simulink model "Model"  (R2020b)
settings: Solver=FixedStepDiscrete  StartTime=0.0  StopTime=inf  RelTol=1e-3
undefined symbols (not defined in the file): C12, designMultirateFIR, dt0
libraries: dspmlti4 x96, dspsrcs4 x89
(part 1 of 6)
settings Model: Creator=User  LastModifiedBy=User

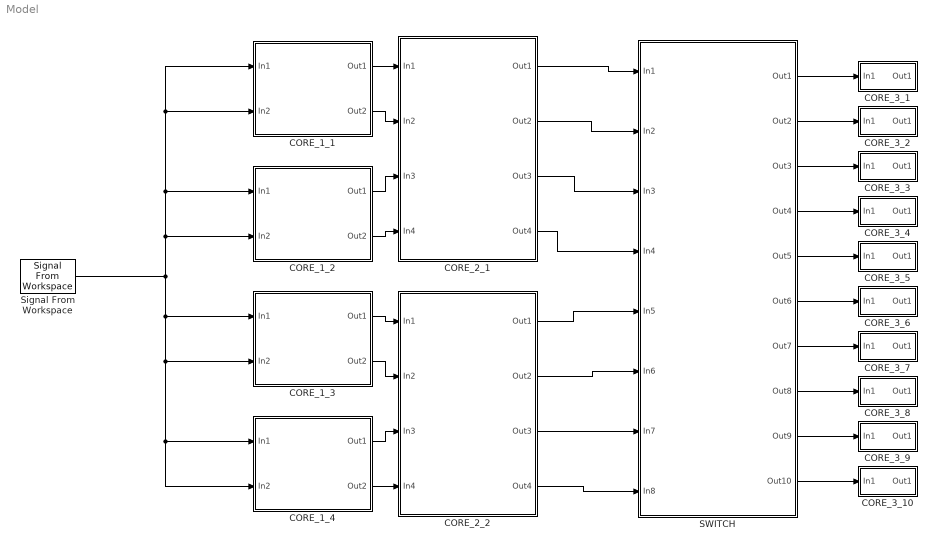
== system Model ==
  CORE_1_1 : Subsystem
  CORE_1_2 : Subsystem
  CORE_1_3 : Subsystem
  CORE_1_4 : Subsystem
  CORE_2_1 : Subsystem
  CORE_2_2 : Subsystem
  CORE_3_1 : Subsystem
  CORE_3_10 : Subsystem
  CORE_3_2 : Subsystem
  CORE_3_3 : Subsystem
  CORE_3_4 : Subsystem
  CORE_3_5 : Subsystem
  CORE_3_6 : Subsystem
  CORE_3_7 : Subsystem
  CORE_3_8 : Subsystem
  CORE_3_9 : Subsystem
  SWITCH : Subsystem
  Signal From Workspace : dspsrcs4/Signal From Workspace  X=x  Ts=dt0  nsamps=1  OutputAfterFinalValue=Cyclic repetition  ignoreOrWarnInputAndFrameLengths=off  OutputFrames=off
  wires:
  CORE_1_4/1(Out1) -> CORE_2_2/3(In3)
  CORE_1_4/2(Out2) -> CORE_2_2/4(In4)
  Signal From Workspace/1 -> CORE_1_2/2(In2), CORE_1_2/1(In1), CORE_1_1/2(In2), CORE_1_1/1(In1), CORE_1_3/1(In1), CORE_1_3/2(In2), CORE_1_4/1(In1), CORE_1_4/2(In2)
  CORE_1_3/2(Out2) -> CORE_2_2/2(In2)
  CORE_1_3/1(Out1) -> CORE_2_2/1(In1)
  CORE_1_1/1(Out1) -> CORE_2_1/1(In1)
  CORE_1_1/2(Out2) -> CORE_2_1/2(In2)
  CORE_1_2/1(Out1) -> CORE_2_1/3(In3)
  CORE_1_2/2(Out2) -> CORE_2_1/4(In4)
  CORE_2_1/1(Out1) -> SWITCH/1(In1)
  CORE_2_1/2(Out2) -> SWITCH/2(In2)
  CORE_2_1/3(Out3) -> SWITCH/3(In3)
  CORE_2_1/4(Out4) -> SWITCH/4(In4)
  CORE_2_2/1(Out1) -> SWITCH/5(In5)
  CORE_2_2/2(Out2) -> SWITCH/6(In6)
  CORE_2_2/3(Out3) -> SWITCH/7(In7)
  CORE_2_2/4(Out4) -> SWITCH/8(In8)
  SWITCH/1(Out1) -> CORE_3_1/1(In1)
  SWITCH/2(Out2) -> CORE_3_2/1(In1)
  SWITCH/3(Out3) -> CORE_3_3/1(In1)
  SWITCH/6(Out6) -> CORE_3_6/1(In1)
  SWITCH/5(Out5) -> CORE_3_5/1(In1)
  SWITCH/4(Out4) -> CORE_3_4/1(In1)
  SWITCH/9(Out9) -> CORE_3_9/1(In1)
  SWITCH/8(Out8) -> CORE_3_8/1(In1)
  SWITCH/7(Out7) -> CORE_3_7/1(In1)
  SWITCH/10(Out10) -> CORE_3_10/1(In1)

== system Model/CORE_1_1 ==
  In1 : Inport
  In2 : Inport  Port=2
  Complex to Real-Imag{,1..3} (4 alike) : ComplexToRealImag
  Constant : Constant  Value=C12  SampleTime=dt0
  Constant1 : Constant  Value=C12  SampleTime=dt0
  DDS_Gen1 : Subsystem
  DDS_Gen2 : Subsystem
  FIR Dec1 : dspmlti4/FIR Decimation  FilterSource=Input port  h=designMultirateFIR(1,2)  D=2  filtStruct=Direct form  FilterObject=FDECIM  framing=Allow multirate processing  inputOffset=0  outputBufInitCond=0  roundingMode=Floor  overflowMode=off  firstCoeffDataTypeStr=Inherit: Same word length as input  firstCoeffMin=[]  firstCoeffMax=[]  firstCoeffLastDataTypeStr=Inherit: Same word length as input  outputDataTypeStr=Inherit: Same as accumulator  outputMin=[]  outputMax=[]  outputLastDataTypeStr=Inherit: Same as accumulator
  FIR Dec2 : dspmlti4/FIR Decimation  FilterSource=Input port  h=designMultirateFIR(1,2)  D=2  filtStruct=Direct form  FilterObject=FDECIM  framing=Allow multirate processing  inputOffset=0  outputBufInitCond=0  roundingMode=Floor  overflowMode=off  firstCoeffDataTypeStr=Inherit: Same word length as input  firstCoeffMin=[]  firstCoeffMax=[]  firstCoeffLastDataTypeStr=Inherit: Same word length as input  outputDataTypeStr=Inherit: Same as accumulator  outputMin=[]  outputMax=[]  outputLastDataTypeStr=Inherit: Same as accumulator
  Freq1 : Constant  Value=-17.5e6
  Freq2 : Constant  Value=-12.5e6
  Mixer1 : Subsystem
  Mixer2 : Subsystem
  Real-Imag to Complex : RealImagToComplex
  Real-Imag to Complex1 : RealImagToComplex
  Out1 : Outport
  Out2 : Outport  Port=2
  wires:
  Complex to Real-Imag/1 -> Mixer1/1(Input_I)
  Complex to Real-Imag/2 -> Mixer1/2(Input_Q)
  Constant1/1 -> FIR Dec2/2
  Mixer2/2(Output_Q) -> Real-Imag to Complex1/2
  Mixer2/1(Output_I) -> Real-Imag to Complex1/1
  Complex to Real-Imag2/1 -> Mixer2/1(Input_I)
  Mixer1/2(Output_Q) -> Real-Imag to Complex/2
  Complex to Real-Imag2/2 -> Mixer2/2(Input_Q)
  Complex to Real-Imag3/1 -> Mixer2/3(DDS_I)
  FIR Dec2/1 -> Out2/1
  Complex to Real-Imag1/1 -> Mixer1/3(DDS_I)
  DDS_Gen1/1(Out1) -> Complex to Real-Imag1/1
  Freq1/1 -> DDS_Gen1/1(In1)
  Complex to Real-Imag1/2 -> Mixer1/4(DDS_Q)
  Real-Imag to Complex1/1 -> FIR Dec2/1
  Complex to Real-Imag3/2 -> Mixer2/4(DDS_Q)
  Freq2/1 -> DDS_Gen2/1(In1)
  DDS_Gen2/1(Out1) -> Complex to Real-Imag3/1
  Real-Imag to Complex/1 -> FIR Dec1/1
  Mixer1/1(Output_I) -> Real-Imag to Complex/1
  Constant/1 -> FIR Dec1/2
  In2/1 -> Complex to Real-Imag2/1
  FIR Dec1/1 -> Out1/1
  In1/1 -> Complex to Real-Imag/1

== system Model/CORE_1_2 ==
  In1 : Inport
  In2 : Inport  Port=2
  Complex to Real-Imag{,1..3} (4 alike) : ComplexToRealImag
  Constant : Constant  Value=C12  SampleTime=dt0
  Constant1 : Constant  Value=C12  SampleTime=dt0
  DDS_Gen1 : Subsystem
  DDS_Gen2 : Subsystem
  FIR Dec1 : dspmlti4/FIR Decimation  FilterSource=Input port  h=designMultirateFIR(1,2)  D=2  filtStruct=Direct form  FilterObject=FDECIM  framing=Allow multirate processing  inputOffset=0  outputBufInitCond=0  roundingMode=Floor  overflowMode=off  firstCoeffDataTypeStr=Inherit: Same word length as input  firstCoeffMin=[]  firstCoeffMax=[]  firstCoeffLastDataTypeStr=Inherit: Same word length as input  outputDataTypeStr=Inherit: Same as accumulator  outputMin=[]  outputMax=[]  outputLastDataTypeStr=Inherit: Same as accumulator
  FIR Dec2 : dspmlti4/FIR Decimation  FilterSource=Input port  h=designMultirateFIR(1,2)  D=2  filtStruct=Direct form  FilterObject=FDECIM  framing=Allow multirate processing  inputOffset=0  outputBufInitCond=0  roundingMode=Floor  overflowMode=off  firstCoeffDataTypeStr=Inherit: Same word length as input  firstCoeffMin=[]  firstCoeffMax=[]  firstCoeffLastDataTypeStr=Inherit: Same word length as input  outputDataTypeStr=Inherit: Same as accumulator  outputMin=[]  outputMax=[]  outputLastDataTypeStr=Inherit: Same as accumulator
  Freq1 : Constant  Value=-7.5e6
  Freq2 : Constant  Value=-2.5e6
  Mixer1 : Subsystem
  Mixer2 : Subsystem
  Real-Imag to Complex : RealImagToComplex
  Real-Imag to Complex1 : RealImagToComplex
  Out1 : Outport
  Out2 : Outport  Port=2
  wires:
  Complex to Real-Imag/1 -> Mixer1/1(Input_I)
  Complex to Real-Imag/2 -> Mixer1/2(Input_Q)
  Constant1/1 -> FIR Dec2/2
  Mixer2/2(Output_Q) -> Real-Imag to Complex1/2
  Mixer2/1(Output_I) -> Real-Imag to Complex1/1
  Complex to Real-Imag2/1 -> Mixer2/1(Input_I)
  Mixer1/2(Output_Q) -> Real-Imag to Complex/2
  Complex to Real-Imag2/2 -> Mixer2/2(Input_Q)
  Complex to Real-Imag3/1 -> Mixer2/3(DDS_I)
  FIR Dec2/1 -> Out2/1
  Complex to Real-Imag1/1 -> Mixer1/3(DDS_I)
  DDS_Gen1/1(Out1) -> Complex to Real-Imag1/1
  Freq1/1 -> DDS_Gen1/1(In1)
  Complex to Real-Imag1/2 -> Mixer1/4(DDS_Q)
  Real-Imag to Complex1/1 -> FIR Dec2/1
  Complex to Real-Imag3/2 -> Mixer2/4(DDS_Q)
  Freq2/1 -> DDS_Gen2/1(In1)
  DDS_Gen2/1(Out1) -> Complex to Real-Imag3/1
  Real-Imag to Complex/1 -> FIR Dec1/1
  Mixer1/1(Output_I) -> Real-Imag to Complex/1
  Constant/1 -> FIR Dec1/2
  In2/1 -> Complex to Real-Imag2/1
  FIR Dec1/1 -> Out1/1
  In1/1 -> Complex to Real-Imag/1

== system Model/CORE_1_3 ==
  In1 : Inport
  In2 : Inport  Port=2
  Complex to Real-Imag{,1..3} (4 alike) : ComplexToRealImag
  Constant : Constant  Value=C12  SampleTime=dt0
  Constant1 : Constant  Value=C12  SampleTime=dt0
  DDS_Gen1 : Subsystem
  DDS_Gen2 : Subsystem
  FIR Dec1 : dspmlti4/FIR Decimation  FilterSource=Input port  h=designMultirateFIR(1,2)  D=2  filtStruct=Direct form  FilterObject=FDECIM  framing=Allow multirate processing  inputOffset=0  outputBufInitCond=0  roundingMode=Floor  overflowMode=off  firstCoeffDataTypeStr=Inherit: Same word length as input  firstCoeffMin=[]  firstCoeffMax=[]  firstCoeffLastDataTypeStr=Inherit: Same word length as input  outputDataTypeStr=Inherit: Same as accumulator  outputMin=[]  outputMax=[]  outputLastDataTypeStr=Inherit: Same as accumulator
  FIR Dec2 : dspmlti4/FIR Decimation  FilterSource=Input port  h=designMultirateFIR(1,2)  D=2  filtStruct=Direct form  FilterObject=FDECIM  framing=Allow multirate processing  inputOffset=0  outputBufInitCond=0  roundingMode=Floor  overflowMode=off  firstCoeffDataTypeStr=Inherit: Same word length as input  firstCoeffMin=[]  firstCoeffMax=[]  firstCoeffLastDataTypeStr=Inherit: Same word length as input  outputDataTypeStr=Inherit: Same as accumulator  outputMin=[]  outputMax=[]  outputLastDataTypeStr=Inherit: Same as accumulator
  Freq1 : Constant  Value=2.5e6
  Freq2 : Constant  Value=7.5e6
  Mixer1 : Subsystem
  Mixer2 : Subsystem
  Real-Imag to Complex : RealImagToComplex
  Real-Imag to Complex1 : RealImagToComplex
  Out1 : Outport
  Out2 : Outport  Port=2
  wires:
  Complex to Real-Imag/1 -> Mixer1/1(Input_I)
  Complex to Real-Imag/2 -> Mixer1/2(Input_Q)
  Constant1/1 -> FIR Dec2/2
  Mixer2/2(Output_Q) -> Real-Imag to Complex1/2
  Mixer2/1(Output_I) -> Real-Imag to Complex1/1
  Complex to Real-Imag2/1 -> Mixer2/1(Input_I)
  Mixer1/2(Output_Q) -> Real-Imag to Complex/2
  Complex to Real-Imag2/2 -> Mixer2/2(Input_Q)
  Complex to Real-Imag3/1 -> Mixer2/3(DDS_I)
  FIR Dec2/1 -> Out2/1
  Complex to Real-Imag1/1 -> Mixer1/3(DDS_I)
  DDS_Gen1/1(Out1) -> Complex to Real-Imag1/1
  Freq1/1 -> DDS_Gen1/1(In1)
  Complex to Real-Imag1/2 -> Mixer1/4(DDS_Q)
  Real-Imag to Complex1/1 -> FIR Dec2/1
  Complex to Real-Imag3/2 -> Mixer2/4(DDS_Q)
  Freq2/1 -> DDS_Gen2/1(In1)
  DDS_Gen2/1(Out1) -> Complex to Real-Imag3/1
  Real-Imag to Complex/1 -> FIR Dec1/1
  Mixer1/1(Output_I) -> Real-Imag to Complex/1
  Constant/1 -> FIR Dec1/2
  In2/1 -> Complex to Real-Imag2/1
  FIR Dec1/1 -> Out1/1
  In1/1 -> Complex to Real-Imag/1

== system Model/CORE_1_4 ==
  In1 : Inport
  In2 : Inport  Port=2
  Complex to Real-Imag{,1..3} (4 alike) : ComplexToRealImag
  Constant : Constant  Value=C12  SampleTime=dt0
  Constant1 : Constant  Value=C12  SampleTime=dt0
  DDS_Gen1 : Subsystem
  DDS_Gen2 : Subsystem
  FIR Dec1 : dspmlti4/FIR Decimation  FilterSource=Input port  h=designMultirateFIR(1,2)  D=2  filtStruct=Direct form  FilterObject=FDECIM  framing=Allow multirate processing  inputOffset=0  outputBufInitCond=0  roundingMode=Floor  overflowMode=off  firstCoeffDataTypeStr=Inherit: Same word length as input  firstCoeffMin=[]  firstCoeffMax=[]  firstCoeffLastDataTypeStr=Inherit: Same word length as input  outputDataTypeStr=Inherit: Same as accumulator  outputMin=[]  outputMax=[]  outputLastDataTypeStr=Inherit: Same as accumulator
  FIR Dec2 : dspmlti4/FIR Decimation  FilterSource=Input port  h=designMultirateFIR(1,2)  D=2  filtStruct=Direct form  FilterObject=FDECIM  framing=Allow multirate processing  inputOffset=0  outputBufInitCond=0  roundingMode=Floor  overflowMode=off  firstCoeffDataTypeStr=Inherit: Same word length as input  firstCoeffMin=[]  firstCoeffMax=[]  firstCoeffLastDataTypeStr=Inherit: Same word length as input  outputDataTypeStr=Inherit: Same as accumulator  outputMin=[]  outputMax=[]  outputLastDataTypeStr=Inherit: Same as accumulator
  Freq1 : Constant  Value=12.5e6
  Freq2 : Constant  Value=17.5e6
  Mixer1 : Subsystem
  Mixer2 : Subsystem
  Real-Imag to Complex : RealImagToComplex
  Real-Imag to Complex1 : RealImagToComplex
  Out1 : Outport
  Out2 : Outport  Port=2
  wires:
  Complex to Real-Imag/1 -> Mixer1/1(Input_I)
  Complex to Real-Imag/2 -> Mixer1/2(Input_Q)
  Constant1/1 -> FIR Dec2/2
  Mixer2/2(Output_Q) -> Real-Imag to Complex1/2
  Mixer2/1(Output_I) -> Real-Imag to Complex1/1
  Complex to Real-Imag2/1 -> Mixer2/1(Input_I)
  Mixer1/2(Output_Q) -> Real-Imag to Complex/2
  Complex to Real-Imag2/2 -> Mixer2/2(Input_Q)
  Complex to Real-Imag3/1 -> Mixer2/3(DDS_I)
  FIR Dec2/1 -> Out2/1
  Complex to Real-Imag1/1 -> Mixer1/3(DDS_I)
  DDS_Gen1/1(Out1) -> Complex to Real-Imag1/1
  Freq1/1 -> DDS_Gen1/1(In1)
  Complex to Real-Imag1/2 -> Mixer1/4(DDS_Q)
  Real-Imag to Complex1/1 -> FIR Dec2/1
  Complex to Real-Imag3/2 -> Mixer2/4(DDS_Q)
  Freq2/1 -> DDS_Gen2/1(In1)
  DDS_Gen2/1(Out1) -> Complex to Real-Imag3/1
  Real-Imag to Complex/1 -> FIR Dec1/1
  Mixer1/1(Output_I) -> Real-Imag to Complex/1
  Constant/1 -> FIR Dec1/2
  In2/1 -> Complex to Real-Imag2/1
  FIR Dec1/1 -> Out1/1
  In1/1 -> Complex to Real-Imag/1

== system Model/CORE_2_1 ==
  In1 : Inport
  In2 : Inport  Port=2
  In3 : Inport  Port=3
  In4 : Inport  Port=4
  Constant{,1..3} (4 alike) : Constant  Value=C12  SampleTime=dt0
  FIR Dec{1..4} (4 alike) : dspmlti4/FIR Decimation  FilterSource=Input port  h=designMultirateFIR(1,2)  D=2  filtStruct=Direct form  FilterObject=FDECIM  framing=Allow multirate processing  inputOffset=0  outputBufInitCond=0  roundingMode=Floor  overflowMode=off  firstCoeffDataTypeStr=Inherit: Same word length as input  firstCoeffMin=[]  firstCoeffMax=[]  firstCoeffLastDataTypeStr=Inherit: Same word length as input  outputDataTypeStr=Inherit: Same as accumulator  outputMin=[]  outputMax=[]  outputLastDataTypeStr=Inherit: Same as accumulator
  Out1 : Outport
  Out2 : Outport  Port=2
  Out3 : Outport  Port=3
  Out4 : Outport  Port=4
  wires:
  Constant1/1 -> FIR Dec2/2
  In1/1 -> FIR Dec1/1
  In4/1 -> FIR Dec4/1
  Constant/1 -> FIR Dec1/2
  Constant2/1 -> FIR Dec3/2
  FIR Dec3/1 -> Out3/1
  Constant3/1 -> FIR Dec4/2
  In2/1 -> FIR Dec2/1
  In3/1 -> FIR Dec3/1
  FIR Dec4/1 -> Out4/1
  FIR Dec1/1 -> Out1/1
  FIR Dec2/1 -> Out2/1

== system Model/CORE_2_2 ==
  In1 : Inport
  In2 : Inport  Port=2
  In3 : Inport  Port=3
  In4 : Inport  Port=4
  Constant{,1..3} (4 alike) : Constant  Value=C12  SampleTime=dt0
  FIR Dec{1..4} (4 alike) : dspmlti4/FIR Decimation  FilterSource=Input port  h=designMultirateFIR(1,2)  D=2  filtStruct=Direct form  FilterObject=FDECIM  framing=Allow multirate processing  inputOffset=0  outputBufInitCond=0  roundingMode=Floor  overflowMode=off  firstCoeffDataTypeStr=Inherit: Same word length as input  firstCoeffMin=[]  firstCoeffMax=[]  firstCoeffLastDataTypeStr=Inherit: Same word length as input  outputDataTypeStr=Inherit: Same as accumulator  outputMin=[]  outputMax=[]  outputLastDataTypeStr=Inherit: Same as accumulator
  Out1 : Outport
  Out2 : Outport  Port=2
  Out3 : Outport  Port=3
  Out4 : Outport  Port=4
  wires:
  Constant1/1 -> FIR Dec2/2
  In1/1 -> FIR Dec1/1
  In4/1 -> FIR Dec4/1
  Constant/1 -> FIR Dec1/2
  Constant2/1 -> FIR Dec3/2
  FIR Dec3/1 -> Out3/1
  Constant3/1 -> FIR Dec4/2
  In2/1 -> FIR Dec2/1
  In3/1 -> FIR Dec3/1
  FIR Dec4/1 -> Out4/1
  FIR Dec1/1 -> Out1/1
  FIR Dec2/1 -> Out2/1

== system Model/CORE_3_1 ==
  In1 : Inport
  Bus Creator4 : BusCreator  Inputs=8
  Bus Selector : BusSelector  OutputSignals=signal1,signal2,signal3,signal4,signal5,signal6,signal7,signal8
  Path1 : Subsystem
  Path2 : Subsystem
  Path3 : Subsystem
  Path4 : Subsystem
  Path5 : Subsystem
  Path6 : Subsystem
  Path7 : Subsystem
  Path8 : Subsystem
  Out1 : Outport
  wires:
  Bus Selector/2 -> Path2/1(<IQ>)  "<signal2>"
  Path8/1(Out1) -> Bus Creator4/8
  Bus Selector/3 -> Path3/1(<IQ>)  "<signal3>"
  Path6/1(Out1) -> Bus Creator4/6
  Bus Selector/6 -> Path6/1(<IQ>)  "<signal6>"
  Bus Selector/4 -> Path4/1(<IQ>)  "<signal4>"
  Path7/1(Out1) -> Bus Creator4/7
  Bus Selector/7 -> Path7/1(<IQ>)  "<signal7>"
  Bus Creator4/1 -> Out1/1
  Path1/1(Out1) -> Bus Creator4/1
  Bus Selector/1 -> Path1/1(<IQ>)  "<signal1>"
  Bus Selector/8 -> Path8/1(<IQ>)  "<signal8>"
  Path3/1(Out1) -> Bus Creator4/3
  Path4/1(Out1) -> Bus Creator4/4
  Path5/1(Out1) -> Bus Creator4/5
  Bus Selector/5 -> Path5/1(<IQ>)  "<signal5>"
  Path2/1(Out1) -> Bus Creator4/2
  In1/1 -> Bus Selector/1

== system Model/CORE_3_10 ==
  In1 : Inport
  Bus Creator4 : BusCreator  Inputs=8
  Bus Selector : BusSelector  OutputSignals=signal1,signal2,signal3,signal4,signal5,signal6,signal7,signal8
  Path1 : Subsystem
  Path2 : Subsystem
  Path3 : Subsystem
  Path4 : Subsystem
  Path5 : Subsystem
  Path6 : Subsystem
  Path7 : Subsystem
  Path8 : Subsystem
  Out1 : Outport
  wires:
  Bus Selector/2 -> Path2/1(<IQ>)  "<signal2>"
  Path8/1(Out1) -> Bus Creator4/8
  Bus Selector/3 -> Path3/1(<IQ>)  "<signal3>"
  Path6/1(Out1) -> Bus Creator4/6
  Bus Selector/6 -> Path6/1(<IQ>)  "<signal6>"
  Bus Selector/4 -> Path4/1(<IQ>)  "<signal4>"
  Path7/1(Out1) -> Bus Creator4/7
  Bus Selector/7 -> Path7/1(<IQ>)  "<signal7>"
  Bus Creator4/1 -> Out1/1
  Path1/1(Out1) -> Bus Creator4/1
  Bus Selector/1 -> Path1/1(<IQ>)  "<signal1>"
  Bus Selector/8 -> Path8/1(<IQ>)  "<signal8>"
  Path3/1(Out1) -> Bus Creator4/3
  Path4/1(Out1) -> Bus Creator4/4
  Path5/1(Out1) -> Bus Creator4/5
  Bus Selector/5 -> Path5/1(<IQ>)  "<signal5>"
  Path2/1(Out1) -> Bus Creator4/2
  In1/1 -> Bus Selector/1

== system Model/CORE_3_2 ==
  In1 : Inport
  Bus Creator4 : BusCreator  Inputs=8
  Bus Selector : BusSelector  OutputSignals=signal1,signal2,signal3,signal4,signal5,signal6,signal7,signal8
  Path1 : Subsystem
  Path2 : Subsystem
  Path3 : Subsystem
  Path4 : Subsystem
  Path5 : Subsystem
  Path6 : Subsystem
  Path7 : Subsystem
  Path8 : Subsystem
  Out1 : Outport
  wires:
  Bus Selector/2 -> Path2/1(<IQ>)  "<signal2>"
  Path8/1(Out1) -> Bus Creator4/8
  Bus Selector/3 -> Path3/1(<IQ>)  "<signal3>"
  Path6/1(Out1) -> Bus Creator4/6
  Bus Selector/6 -> Path6/1(<IQ>)  "<signal6>"
  Bus Selector/4 -> Path4/1(<IQ>)  "<signal4>"
  Path7/1(Out1) -> Bus Creator4/7
  Bus Selector/7 -> Path7/1(<IQ>)  "<signal7>"
  Bus Creator4/1 -> Out1/1
  Path1/1(Out1) -> Bus Creator4/1
  Bus Selector/1 -> Path1/1(<IQ>)  "<signal1>"
  Bus Selector/8 -> Path8/1(<IQ>)  "<signal8>"
  Path3/1(Out1) -> Bus Creator4/3
  Path4/1(Out1) -> Bus Creator4/4
  Path5/1(Out1) -> Bus Creator4/5
  Bus Selector/5 -> Path5/1(<IQ>)  "<signal5>"
  Path2/1(Out1) -> Bus Creator4/2
  In1/1 -> Bus Selector/1

== system Model/CORE_3_3 ==
  In1 : Inport
  Bus Creator4 : BusCreator  Inputs=8
  Bus Selector : BusSelector  OutputSignals=signal1,signal2,signal3,signal4,signal5,signal6,signal7,signal8
  Path1 : Subsystem
  Path2 : Subsystem
  Path3 : Subsystem
  Path4 : Subsystem
  Path5 : Subsystem
  Path6 : Subsystem
  Path7 : Subsystem
  Path8 : Subsystem
  Out1 : Outport
  wires:
  Bus Selector/2 -> Path2/1(<IQ>)  "<signal2>"
  Path8/1(Out1) -> Bus Creator4/8
  Bus Selector/3 -> Path3/1(<IQ>)  "<signal3>"
  Path6/1(Out1) -> Bus Creator4/6
  Bus Selector/6 -> Path6/1(<IQ>)  "<signal6>"
  Bus Selector/4 -> Path4/1(<IQ>)  "<signal4>"
  Path7/1(Out1) -> Bus Creator4/7
  Bus Selector/7 -> Path7/1(<IQ>)  "<signal7>"
  Bus Creator4/1 -> Out1/1
  Path1/1(Out1) -> Bus Creator4/1
  Bus Selector/1 -> Path1/1(<IQ>)  "<signal1>"
  Bus Selector/8 -> Path8/1(<IQ>)  "<signal8>"
  Path3/1(Out1) -> Bus Creator4/3
  Path4/1(Out1) -> Bus Creator4/4
  Path5/1(Out1) -> Bus Creator4/5
  Bus Selector/5 -> Path5/1(<IQ>)  "<signal5>"
  Path2/1(Out1) -> Bus Creator4/2
  In1/1 -> Bus Selector/1

== system Model/CORE_3_4 ==
  In1 : Inport
  Bus Creator4 : BusCreator  Inputs=8
  Bus Selector : BusSelector  OutputSignals=signal1,signal2,signal3,signal4,signal5,signal6,signal7,signal8
  Path1 : Subsystem
  Path2 : Subsystem
  Path3 : Subsystem
  Path4 : Subsystem
  Path5 : Subsystem
  Path6 : Subsystem
  Path7 : Subsystem
  Path8 : Subsystem
  Out1 : Outport
  wires:
  Bus Selector/2 -> Path2/1(<IQ>)  "<signal2>"
  Path8/1(Out1) -> Bus Creator4/8
  Bus Selector/3 -> Path3/1(<IQ>)  "<signal3>"
  Path6/1(Out1) -> Bus Creator4/6
  Bus Selector/6 -> Path6/1(<IQ>)  "<signal6>"
  Bus Selector/4 -> Path4/1(<IQ>)  "<signal4>"
  Path7/1(Out1) -> Bus Creator4/7
  Bus Selector/7 -> Path7/1(<IQ>)  "<signal7>"
  Bus Creator4/1 -> Out1/1
  Path1/1(Out1) -> Bus Creator4/1
  Bus Selector/1 -> Path1/1(<IQ>)  "<signal1>"
  Bus Selector/8 -> Path8/1(<IQ>)  "<signal8>"
  Path3/1(Out1) -> Bus Creator4/3
  Path4/1(Out1) -> Bus Creator4/4
  Path5/1(Out1) -> Bus Creator4/5
  Bus Selector/5 -> Path5/1(<IQ>)  "<signal5>"
  Path2/1(Out1) -> Bus Creator4/2
  In1/1 -> Bus Selector/1

== system Model/CORE_3_5 ==
  In1 : Inport
  Bus Creator4 : BusCreator  Inputs=8
  Bus Selector : BusSelector  OutputSignals=signal1,signal2,signal3,signal4,signal5,signal6,signal7,signal8
  Path1 : Subsystem
  Path2 : Subsystem
  Path3 : Subsystem
  Path4 : Subsystem
  Path5 : Subsystem
  Path6 : Subsystem
  Path7 : Subsystem
  Path8 : Subsystem
  Out1 : Outport
  wires:
  Bus Selector/2 -> Path2/1(<IQ>)  "<signal2>"
  Path8/1(Out1) -> Bus Creator4/8
  Bus Selector/3 -> Path3/1(<IQ>)  "<signal3>"
  Path6/1(Out1) -> Bus Creator4/6
  Bus Selector/6 -> Path6/1(<IQ>)  "<signal6>"
  Bus Selector/4 -> Path4/1(<IQ>)  "<signal4>"
  Path7/1(Out1) -> Bus Creator4/7
  Bus Selector/7 -> Path7/1(<IQ>)  "<signal7>"
  Bus Creator4/1 -> Out1/1
  Path1/1(Out1) -> Bus Creator4/1
  Bus Selector/1 -> Path1/1(<IQ>)  "<signal1>"
  Bus Selector/8 -> Path8/1(<IQ>)  "<signal8>"
  Path3/1(Out1) -> Bus Creator4/3
  Path4/1(Out1) -> Bus Creator4/4
  Path5/1(Out1) -> Bus Creator4/5
  Bus Selector/5 -> Path5/1(<IQ>)  "<signal5>"
  Path2/1(Out1) -> Bus Creator4/2
  In1/1 -> Bus Selector/1

== system Model/CORE_3_6 ==
  In1 : Inport
  Bus Creator4 : BusCreator  Inputs=8
  Bus Selector : BusSelector  OutputSignals=signal1,signal2,signal3,signal4,signal5,signal6,signal7,signal8
  Path1 : Subsystem
  Path2 : Subsystem
  Path3 : Subsystem
  Path4 : Subsystem
  Path5 : Subsystem
  Path6 : Subsystem
  Path7 : Subsystem
  Path8 : Subsystem
  Out1 : Outport
  wires:
  Bus Selector/2 -> Path2/1(<IQ>)  "<signal2>"
  Path8/1(Out1) -> Bus Creator4/8
  Bus Selector/3 -> Path3/1(<IQ>)  "<signal3>"
  Path6/1(Out1) -> Bus Creator4/6
  Bus Selector/6 -> Path6/1(<IQ>)  "<signal6>"
  Bus Selector/4 -> Path4/1(<IQ>)  "<signal4>"
  Path7/1(Out1) -> Bus Creator4/7
  Bus Selector/7 -> Path7/1(<IQ>)  "<signal7>"
  Bus Creator4/1 -> Out1/1
  Path1/1(Out1) -> Bus Creator4/1
  Bus Selector/1 -> Path1/1(<IQ>)  "<signal1>"
  Bus Selector/8 -> Path8/1(<IQ>)  "<signal8>"
  Path3/1(Out1) -> Bus Creator4/3
  Path4/1(Out1) -> Bus Creator4/4
  Path5/1(Out1) -> Bus Creator4/5
  Bus Selector/5 -> Path5/1(<IQ>)  "<signal5>"
  Path2/1(Out1) -> Bus Creator4/2
  In1/1 -> Bus Selector/1

== system Model/CORE_3_7 ==
  In1 : Inport
  Bus Creator4 : BusCreator  Inputs=8
  Bus Selector : BusSelector  OutputSignals=signal1,signal2,signal3,signal4,signal5,signal6,signal7,signal8
  Path1 : Subsystem
  Path2 : Subsystem
  Path3 : Subsystem
  Path4 : Subsystem
  Path5 : Subsystem
  Path6 : Subsystem
  Path7 : Subsystem
  Path8 : Subsystem
  Out1 : Outport
  wires:
  Bus Selector/2 -> Path2/1(<IQ>)  "<signal2>"
  Path8/1(Out1) -> Bus Creator4/8
  Bus Selector/3 -> Path3/1(<IQ>)  "<signal3>"
  Path6/1(Out1) -> Bus Creator4/6
  Bus Selector/6 -> Path6/1(<IQ>)  "<signal6>"
  Bus Selector/4 -> Path4/1(<IQ>)  "<signal4>"
  Path7/1(Out1) -> Bus Creator4/7
  Bus Selector/7 -> Path7/1(<IQ>)  "<signal7>"
  Bus Creator4/1 -> Out1/1
  Path1/1(Out1) -> Bus Creator4/1
  Bus Selector/1 -> Path1/1(<IQ>)  "<signal1>"
  Bus Selector/8 -> Path8/1(<IQ>)  "<signal8>"
  Path3/1(Out1) -> Bus Creator4/3
  Path4/1(Out1) -> Bus Creator4/4
  Path5/1(Out1) -> Bus Creator4/5
  Bus Selector/5 -> Path5/1(<IQ>)  "<signal5>"
  Path2/1(Out1) -> Bus Creator4/2
  In1/1 -> Bus Selector/1

== system Model/CORE_3_8 ==
  In1 : Inport
  Bus Creator4 : BusCreator  Inputs=8
  Bus Selector : BusSelector  OutputSignals=signal1,signal2,signal3,signal4,signal5,signal6,signal7,signal8
  Path1 : Subsystem
  Path2 : Subsystem
  Path3 : Subsystem
  Path4 : Subsystem
  Path5 : Subsystem
  Path6 : Subsystem
  Path7 : Subsystem
  Path8 : Subsystem
  Out1 : Outport
  wires:
  Bus Selector/2 -> Path2/1(<IQ>)  "<signal2>"
  Path8/1(Out1) -> Bus Creator4/8
  Bus Selector/3 -> Path3/1(<IQ>)  "<signal3>"
  Path6/1(Out1) -> Bus Creator4/6
  Bus Selector/6 -> Path6/1(<IQ>)  "<signal6>"
  Bus Selector/4 -> Path4/1(<IQ>)  "<signal4>"
  Path7/1(Out1) -> Bus Creator4/7
  Bus Selector/7 -> Path7/1(<IQ>)  "<signal7>"
  Bus Creator4/1 -> Out1/1
  Path1/1(Out1) -> Bus Creator4/1
  Bus Selector/1 -> Path1/1(<IQ>)  "<signal1>"
  Bus Selector/8 -> Path8/1(<IQ>)  "<signal8>"
  Path3/1(Out1) -> Bus Creator4/3
  Path4/1(Out1) -> Bus Creator4/4
  Path5/1(Out1) -> Bus Creator4/5
  Bus Selector/5 -> Path5/1(<IQ>)  "<signal5>"
  Path2/1(Out1) -> Bus Creator4/2
  In1/1 -> Bus Selector/1

== system Model/CORE_3_9 ==
  In1 : Inport
  Bus Creator4 : BusCreator  Inputs=8
  Bus Selector : BusSelector  OutputSignals=signal1,signal2,signal3,signal4,signal5,signal6,signal7,signal8
  Path1 : Subsystem
  Path2 : Subsystem
  Path3 : Subsystem
  Path4 : Subsystem
  Path5 : Subsystem
  Path6 : Subsystem
  Path7 : Subsystem
  Path8 : Subsystem
  Out1 : Outport
  wires:
  Bus Selector/2 -> Path2/1(<IQ>)  "<signal2>"
  Path8/1(Out1) -> Bus Creator4/8
  Bus Selector/3 -> Path3/1(<IQ>)  "<signal3>"
  Path6/1(Out1) -> Bus Creator4/6
  Bus Selector/6 -> Path6/1(<IQ>)  "<signal6>"
  Bus Selector/4 -> Path4/1(<IQ>)  "<signal4>"
  Path7/1(Out1) -> Bus Creator4/7
  Bus Selector/7 -> Path7/1(<IQ>)  "<signal7>"
  Bus Creator4/1 -> Out1/1
  Path1/1(Out1) -> Bus Creator4/1
  Bus Selector/1 -> Path1/1(<IQ>)  "<signal1>"
  Bus Selector/8 -> Path8/1(<IQ>)  "<signal8>"
  Path3/1(Out1) -> Bus Creator4/3
  Path4/1(Out1) -> Bus Creator4/4
  Path5/1(Out1) -> Bus Creator4/5
  Bus Selector/5 -> Path5/1(<IQ>)  "<signal5>"
  Path2/1(Out1) -> Bus Creator4/2
  In1/1 -> Bus Selector/1

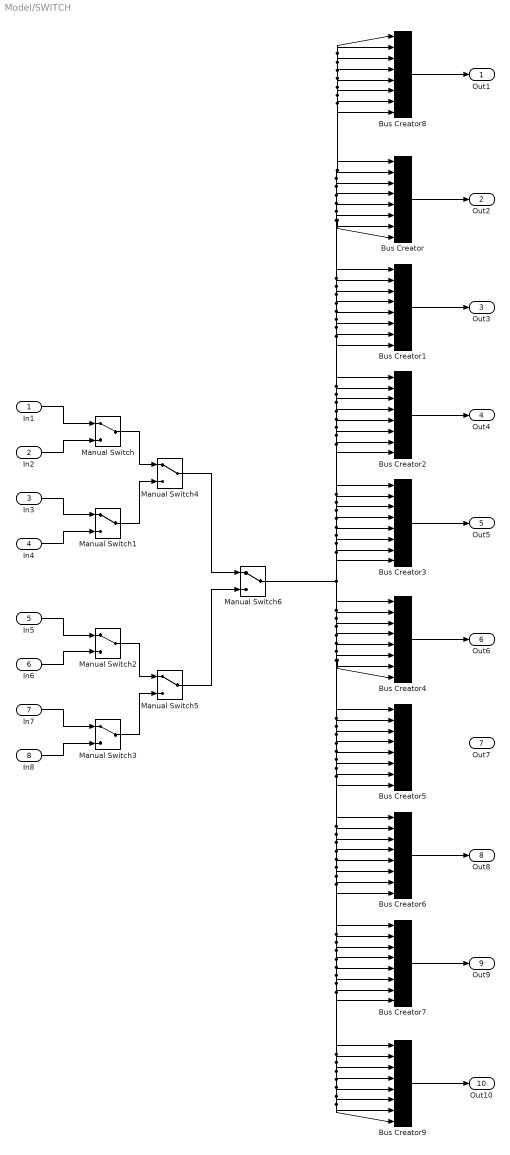
== system Model/SWITCH ==
  In1 : Inport
  In2 : Inport  Port=2
  In3 : Inport  Port=3
  In4 : Inport  Port=4
  In5 : Inport  Port=5
  In6 : Inport  Port=6
  In7 : Inport  Port=7
  In8 : Inport  Port=8
  Bus Creator{,1..9} (10 alike) : BusCreator  Inputs=8
  Manual Switch{,1..6} (7 alike) : ManualSwitch
  Out1 : Outport
  Out2 : Outport  Port=2
  Out3 : Outport  Port=3
  Out4 : Outport  Port=4
  Out5 : Outport  Port=5
  Out6 : Outport  Port=6
  Out7 : Outport  Port=7
  Out8 : Outport  Port=8
  Out9 : Outport  Port=9
  Out10 : Outport  Port=10
  wires:
  Manual Switch/1 -> Manual Switch4/1
  In7/1 -> Manual Switch3/1
  Manual Switch5/1 -> Manual Switch6/2
  In2/1 -> Manual Switch/2
  In4/1 -> Manual Switch1/2
  In1/1 -> Manual Switch/1
  Manual Switch1/1 -> Manual Switch4/2
  Manual Switch3/1 -> Manual Switch5/2
  Manual Switch2/1 -> Manual Switch5/1
  In8/1 -> Manual Switch3/2
  Manual Switch4/1 -> Manual Switch6/1
  In6/1 -> Manual Switch2/2
  In5/1 -> Manual Switch2/1
  In3/1 -> Manual Switch1/1
  Manual Switch6/1 -> Bus Creator9/3, Bus Creator9/4, Bus Creator9/6, Bus Creator9/7, Bus Creator9/8, Bus Creator9/5, Bus Creator9/2, Bus Creator9/1, Bus Creator7/8, Bus Creator7/7, Bus Creator7/6, Bus Creator7/5, Bus Creator7/4, Bus Creator7/3, Bus Creator7/2, Bus Creator7/1, Bus Creator6/8, Bus Creator6/7, Bus Creator6/6, Bus Creator6/5, Bus Creator6/4, Bus Creator6/3, Bus Creator6/2, Bus Creator6/1, Bus Creator5/8, Bus Creator5/7, Bus Creator5/6, Bus Creator5/5, Bus Creator5/4, Bus Creator5/3, Bus Creator5/2, Bus Creator5/1, Bus Creator4/8, Bus Creator4/7, Bus Creator4/6, Bus Creator4/5, Bus Creator4/4, Bus Creator4/3, Bus Creator4/2, Bus Creator4/1, Bus Creator3/8, Bus Creator3/7, Bus Creator3/6, Bus Creator3/5, Bus Creator3/4, Bus Creator3/3, Bus Creator3/2, Bus Creator3/1, Bus Creator2/8, Bus Creator2/7, Bus Creator2/6, Bus Creator2/5, Bus Creator2/4, Bus Creator2/3, Bus Creator2/1, Bus Creator1/8, Bus Creator1/7, Bus Creator1/6, Bus Creator1/5, Bus Creator1/4, Bus Creator1/3, Bus Creator1/2, Bus Creator1/1, Bus Creator8/6, Bus Creator8/5, Bus Creator8/2, Bus Creator8/1, Bus Creator8/3, Bus Creator8/4, Bus Creator8/7, Bus Creator8/8, Bus Creator/1, Bus Creator/2, Bus Creator/3, Bus Creator/4, Bus Creator/5, Bus Creator/6, Bus Creator/8, Bus Creator/7, Bus Creator2/2
  Bus Creator8/1 -> Out1/1
  Bus Creator/1 -> Out2/1
  Bus Creator1/1 -> Out3/1
  Bus Creator2/1 -> Out4/1
  Bus Creator3/1 -> Out5/1
  ? -> Out7/1
  Bus Creator6/1 -> Out8/1
  Bus Creator4/1 -> Out6/1
  Bus Creator7/1 -> Out9/1
  Bus Creator9/1 -> Out10/1

== system Model/CORE_1_1/DDS_Gen1 ==
  In1 : Inport
  Exp : Math  SaturateOnIntegerOverflow=on
  Gain : Gain  Gain=-1i*2*pi
  Product : Product
  Signal From Workspace1 : dspsrcs4/Signal From Workspace  X=t0  Ts=dt0  nsamps=1  OutputAfterFinalValue=Cyclic repetition  ignoreOrWarnInputAndFrameLengths=off  OutputFrames=off
  Out1 : Outport
  wires:
  Signal From Workspace1/1 -> Gain/1
  Exp/1 -> Out1/1
  Gain/1 -> Product/2
  Product/1 -> Exp/1
  In1/1 -> Product/1

== system Model/CORE_1_1/DDS_Gen2 ==
  In1 : Inport
  Exp : Math  SaturateOnIntegerOverflow=on
  Gain : Gain  Gain=-1i*2*pi
  Product : Product
  Signal From Workspace1 : dspsrcs4/Signal From Workspace  X=t0  Ts=dt0  nsamps=1  OutputAfterFinalValue=Cyclic repetition  ignoreOrWarnInputAndFrameLengths=off  OutputFrames=off
  Out1 : Outport
  wires:
  Signal From Workspace1/1 -> Gain/1
  Exp/1 -> Out1/1
  Gain/1 -> Product/2
  Product/1 -> Exp/1
  In1/1 -> Product/1

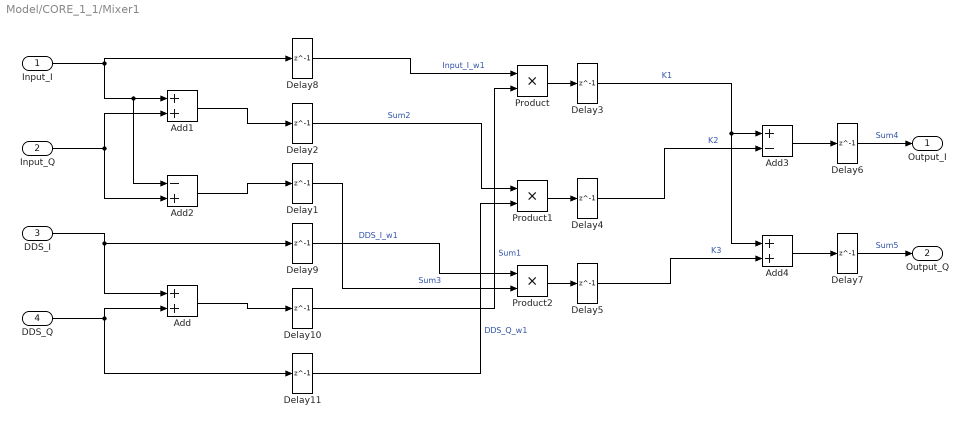
== system Model/CORE_1_1/Mixer1 ==
  Input_I : Inport
  Input_Q : Inport  Port=2
  DDS_I : Inport  Port=3
  DDS_Q : Inport  Port=4
  Add : Sum
  Add1 : Sum
  Add2 : Sum  Inputs=-+
  Add3 : Sum  Inputs=+-
  Add4 : Sum
  Delay{1..11} (11 alike) : Delay  DelayLength=1  InitialCondition=0  SampleTime=dt0
  Product : Product
  Product1 : Product
  Product2 : Product
  Output_I : Outport
  Output_Q : Outport  Port=2
  wires:
  DDS_I/1 -> Delay9/1, Add/1
  Input_Q/1 -> Add2/2, Add1/2
  Add/1 -> Delay10/1
  Delay10/1 -> Product/2  "Sum1"
  Add2/1 -> Delay1/1
  Add1/1 -> Delay2/1
  Product/1 -> Delay3/1
  Delay3/1 -> Add4/1, Add3/1  "K1"
  Delay2/1 -> Product1/1  "Sum2"
  Product1/1 -> Delay4/1
  Delay4/1 -> Add3/2  "K2"
  Delay1/1 -> Product2/2  "Sum3"
  Product2/1 -> Delay5/1
  Delay5/1 -> Add4/2  "K3"
  Add3/1 -> Delay6/1
  Add4/1 -> Delay7/1
  Delay6/1 -> Output_I/1  "Sum4"
  Delay7/1 -> Output_Q/1  "Sum5"
  Input_I/1 -> Add2/1, Add1/1, Delay8/1
  DDS_Q/1 -> Delay11/1, Add/2
  Delay8/1 -> Product/1  "Input_I_w1"
  Delay11/1 -> Product1/2  "DDS_Q_w1"
  Delay9/1 -> Product2/1  "DDS_I_w1"

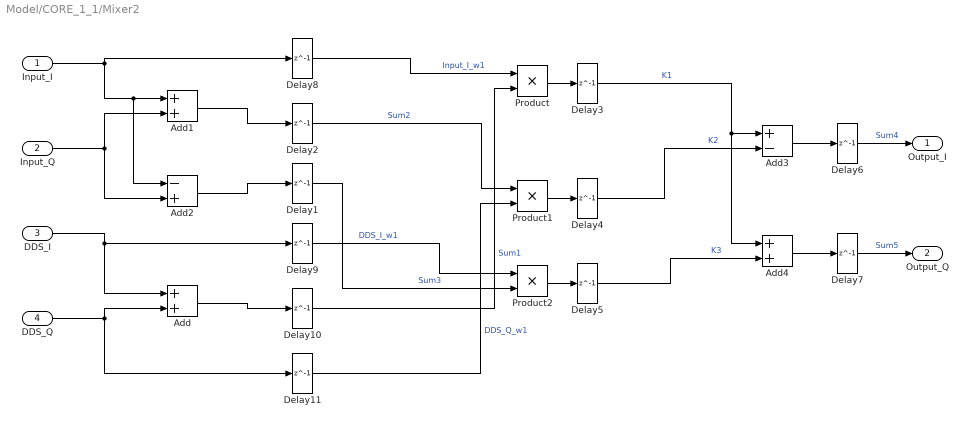
== system Model/CORE_1_1/Mixer2 ==
  Input_I : Inport
  Input_Q : Inport  Port=2
  DDS_I : Inport  Port=3
  DDS_Q : Inport  Port=4
  Add : Sum
  Add1 : Sum
  Add2 : Sum  Inputs=-+
  Add3 : Sum  Inputs=+-
  Add4 : Sum
  Delay{1..11} (11 alike) : Delay  DelayLength=1  InitialCondition=0  SampleTime=dt0
  Product : Product
  Product1 : Product
  Product2 : Product
  Output_I : Outport
  Output_Q : Outport  Port=2
  wires:
  DDS_I/1 -> Delay9/1, Add/1
  Input_Q/1 -> Add2/2, Add1/2
  Add/1 -> Delay10/1
  Delay10/1 -> Product/2  "Sum1"
  Add2/1 -> Delay1/1
  Add1/1 -> Delay2/1
  Product/1 -> Delay3/1
  Delay3/1 -> Add4/1, Add3/1  "K1"
  Delay2/1 -> Product1/1  "Sum2"
  Product1/1 -> Delay4/1
  Delay4/1 -> Add3/2  "K2"
  Delay1/1 -> Product2/2  "Sum3"
  Product2/1 -> Delay5/1
  Delay5/1 -> Add4/2  "K3"
  Add3/1 -> Delay6/1
  Add4/1 -> Delay7/1
  Delay6/1 -> Output_I/1  "Sum4"
  Delay7/1 -> Output_Q/1  "Sum5"
  Input_I/1 -> Add2/1, Add1/1, Delay8/1
  DDS_Q/1 -> Delay11/1, Add/2
  Delay8/1 -> Product/1  "Input_I_w1"
  Delay11/1 -> Product1/2  "DDS_Q_w1"
  Delay9/1 -> Product2/1  "DDS_I_w1"

== system Model/CORE_1_2/DDS_Gen1 ==
  In1 : Inport
  Exp : Math  SaturateOnIntegerOverflow=on
  Gain : Gain  Gain=-1i*2*pi
  Product : Product
  Signal From Workspace1 : dspsrcs4/Signal From Workspace  X=t0  Ts=dt0  nsamps=1  OutputAfterFinalValue=Cyclic repetition  ignoreOrWarnInputAndFrameLengths=off  OutputFrames=off
  Out1 : Outport
  wires:
  Signal From Workspace1/1 -> Gain/1
  Exp/1 -> Out1/1
  Gain/1 -> Product/2
  Product/1 -> Exp/1
  In1/1 -> Product/1

== system Model/CORE_1_2/DDS_Gen2 ==
  In1 : Inport
  Exp : Math  SaturateOnIntegerOverflow=on
  Gain : Gain  Gain=-1i*2*pi
  Product : Product
  Signal From Workspace1 : dspsrcs4/Signal From Workspace  X=t0  Ts=dt0  nsamps=1  OutputAfterFinalValue=Cyclic repetition  ignoreOrWarnInputAndFrameLengths=off  OutputFrames=off
  Out1 : Outport
  wires:
  Signal From Workspace1/1 -> Gain/1
  Exp/1 -> Out1/1
  Gain/1 -> Product/2
  Product/1 -> Exp/1
  In1/1 -> Product/1

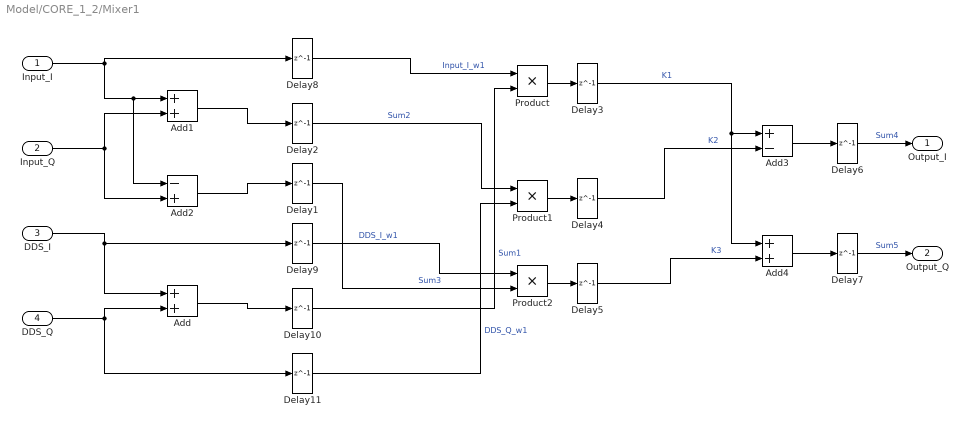
== system Model/CORE_1_2/Mixer1 ==
  Input_I : Inport
  Input_Q : Inport  Port=2
  DDS_I : Inport  Port=3
  DDS_Q : Inport  Port=4
  Add : Sum
  Add1 : Sum
  Add2 : Sum  Inputs=-+
  Add3 : Sum  Inputs=+-
  Add4 : Sum
  Delay{1..11} (11 alike) : Delay  DelayLength=1  InitialCondition=0  SampleTime=dt0
  Product : Product
  Product1 : Product
  Product2 : Product
  Output_I : Outport
  Output_Q : Outport  Port=2
  wires:
  DDS_I/1 -> Delay9/1, Add/1
  Input_Q/1 -> Add2/2, Add1/2
  Add/1 -> Delay10/1
  Delay10/1 -> Product/2  "Sum1"
  Add2/1 -> Delay1/1
  Add1/1 -> Delay2/1
  Product/1 -> Delay3/1
  Delay3/1 -> Add4/1, Add3/1  "K1"
  Delay2/1 -> Product1/1  "Sum2"
  Product1/1 -> Delay4/1
  Delay4/1 -> Add3/2  "K2"
  Delay1/1 -> Product2/2  "Sum3"
  Product2/1 -> Delay5/1
  Delay5/1 -> Add4/2  "K3"
  Add3/1 -> Delay6/1
  Add4/1 -> Delay7/1
  Delay6/1 -> Output_I/1  "Sum4"
  Delay7/1 -> Output_Q/1  "Sum5"
  Input_I/1 -> Add2/1, Add1/1, Delay8/1
  DDS_Q/1 -> Delay11/1, Add/2
  Delay8/1 -> Product/1  "Input_I_w1"
  Delay11/1 -> Product1/2  "DDS_Q_w1"
  Delay9/1 -> Product2/1  "DDS_I_w1"

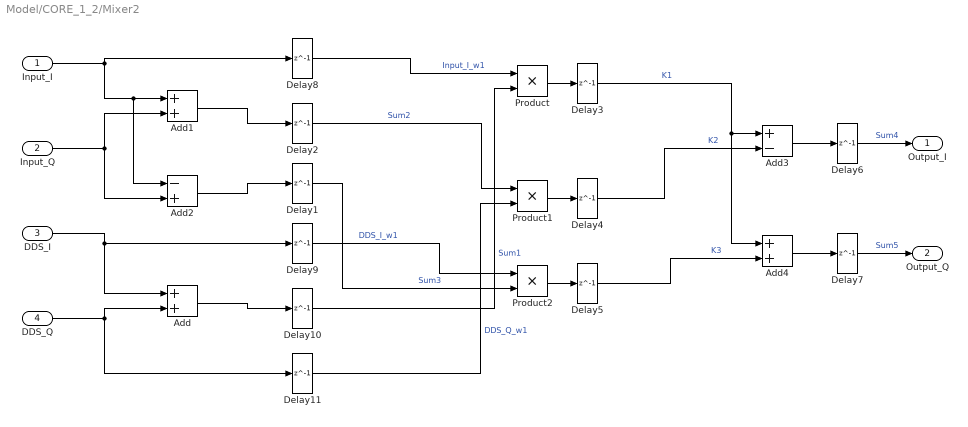
== system Model/CORE_1_2/Mixer2 ==
  Input_I : Inport
  Input_Q : Inport  Port=2
  DDS_I : Inport  Port=3
  DDS_Q : Inport  Port=4
  Add : Sum
  Add1 : Sum
  Add2 : Sum  Inputs=-+
  Add3 : Sum  Inputs=+-
  Add4 : Sum
  Delay{1..11} (11 alike) : Delay  DelayLength=1  InitialCondition=0  SampleTime=dt0
  Product : Product
  Product1 : Product
  Product2 : Product
  Output_I : Outport
  Output_Q : Outport  Port=2
  wires:
  DDS_I/1 -> Delay9/1, Add/1
  Input_Q/1 -> Add2/2, Add1/2
  Add/1 -> Delay10/1
  Delay10/1 -> Product/2  "Sum1"
  Add2/1 -> Delay1/1
  Add1/1 -> Delay2/1
  Product/1 -> Delay3/1
  Delay3/1 -> Add4/1, Add3/1  "K1"
  Delay2/1 -> Product1/1  "Sum2"
  Product1/1 -> Delay4/1
  Delay4/1 -> Add3/2  "K2"
  Delay1/1 -> Product2/2  "Sum3"
  Product2/1 -> Delay5/1
  Delay5/1 -> Add4/2  "K3"
  Add3/1 -> Delay6/1
  Add4/1 -> Delay7/1
  Delay6/1 -> Output_I/1  "Sum4"
  Delay7/1 -> Output_Q/1  "Sum5"
  Input_I/1 -> Add2/1, Add1/1, Delay8/1
  DDS_Q/1 -> Delay11/1, Add/2
  Delay8/1 -> Product/1  "Input_I_w1"
  Delay11/1 -> Product1/2  "DDS_Q_w1"
  Delay9/1 -> Product2/1  "DDS_I_w1"

== system Model/CORE_1_3/DDS_Gen1 ==
  In1 : Inport
  Exp : Math  SaturateOnIntegerOverflow=on
  Gain : Gain  Gain=-1i*2*pi
  Product : Product
  Signal From Workspace1 : dspsrcs4/Signal From Workspace  X=t0  Ts=dt0  nsamps=1  OutputAfterFinalValue=Cyclic repetition  ignoreOrWarnInputAndFrameLengths=off  OutputFrames=off
  Out1 : Outport
  wires:
  Signal From Workspace1/1 -> Gain/1
  Exp/1 -> Out1/1
  Gain/1 -> Product/2
  Product/1 -> Exp/1
  In1/1 -> Product/1

== system Model/CORE_1_3/DDS_Gen2 ==
  In1 : Inport
  Exp : Math  SaturateOnIntegerOverflow=on
  Gain : Gain  Gain=-1i*2*pi
  Product : Product
  Signal From Workspace1 : dspsrcs4/Signal From Workspace  X=t0  Ts=dt0  nsamps=1  OutputAfterFinalValue=Cyclic repetition  ignoreOrWarnInputAndFrameLengths=off  OutputFrames=off
  Out1 : Outport
  wires:
  Signal From Workspace1/1 -> Gain/1
  Exp/1 -> Out1/1
  Gain/1 -> Product/2
  Product/1 -> Exp/1
  In1/1 -> Product/1

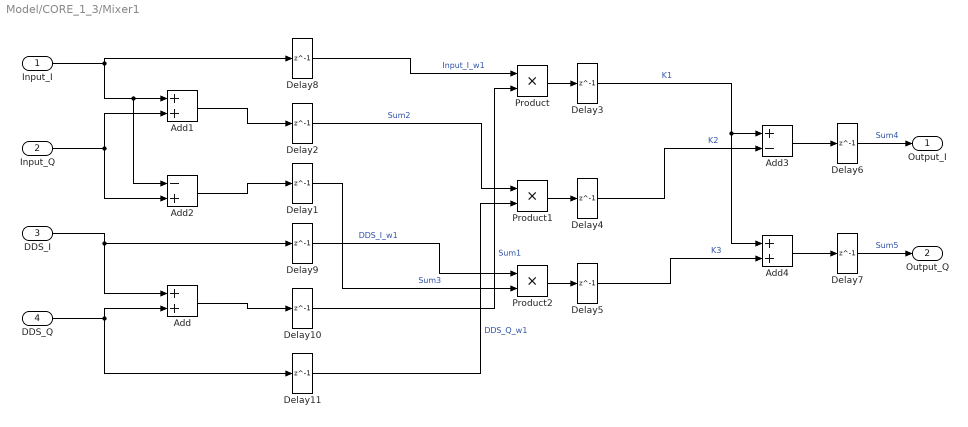
== system Model/CORE_1_3/Mixer1 ==
  Input_I : Inport
  Input_Q : Inport  Port=2
  DDS_I : Inport  Port=3
  DDS_Q : Inport  Port=4
  Add : Sum
  Add1 : Sum
  Add2 : Sum  Inputs=-+
  Add3 : Sum  Inputs=+-
  Add4 : Sum
  Delay{1..11} (11 alike) : Delay  DelayLength=1  InitialCondition=0  SampleTime=dt0
  Product : Product
  Product1 : Product
  Product2 : Product
  Output_I : Outport
  Output_Q : Outport  Port=2
  wires:
  DDS_I/1 -> Delay9/1, Add/1
  Input_Q/1 -> Add2/2, Add1/2
  Add/1 -> Delay10/1
  Delay10/1 -> Product/2  "Sum1"
  Add2/1 -> Delay1/1
  Add1/1 -> Delay2/1
  Product/1 -> Delay3/1
  Delay3/1 -> Add4/1, Add3/1  "K1"
  Delay2/1 -> Product1/1  "Sum2"
  Product1/1 -> Delay4/1
  Delay4/1 -> Add3/2  "K2"
  Delay1/1 -> Product2/2  "Sum3"
  Product2/1 -> Delay5/1
  Delay5/1 -> Add4/2  "K3"
  Add3/1 -> Delay6/1
  Add4/1 -> Delay7/1
  Delay6/1 -> Output_I/1  "Sum4"
  Delay7/1 -> Output_Q/1  "Sum5"
  Input_I/1 -> Add2/1, Add1/1, Delay8/1
  DDS_Q/1 -> Delay11/1, Add/2
  Delay8/1 -> Product/1  "Input_I_w1"
  Delay11/1 -> Product1/2  "DDS_Q_w1"
  Delay9/1 -> Product2/1  "DDS_I_w1"

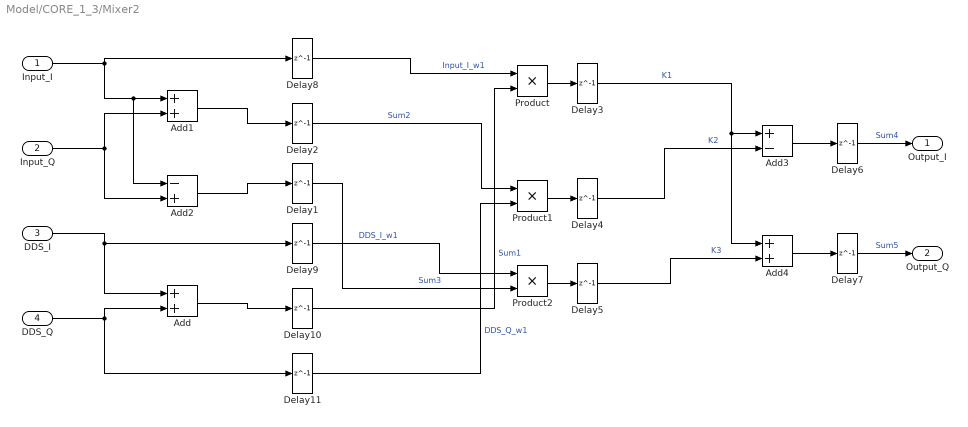
== system Model/CORE_1_3/Mixer2 ==
  Input_I : Inport
  Input_Q : Inport  Port=2
  DDS_I : Inport  Port=3
  DDS_Q : Inport  Port=4
  Add : Sum
  Add1 : Sum
  Add2 : Sum  Inputs=-+
  Add3 : Sum  Inputs=+-
  Add4 : Sum
  Delay{1..11} (11 alike) : Delay  DelayLength=1  InitialCondition=0  SampleTime=dt0
  Product : Product
  Product1 : Product
  Product2 : Product
  Output_I : Outport
  Output_Q : Outport  Port=2
  wires:
  DDS_I/1 -> Delay9/1, Add/1
  Input_Q/1 -> Add2/2, Add1/2
  Add/1 -> Delay10/1
  Delay10/1 -> Product/2  "Sum1"
  Add2/1 -> Delay1/1
  Add1/1 -> Delay2/1
  Product/1 -> Delay3/1
  Delay3/1 -> Add4/1, Add3/1  "K1"
  Delay2/1 -> Product1/1  "Sum2"
  Product1/1 -> Delay4/1
  Delay4/1 -> Add3/2  "K2"
  Delay1/1 -> Product2/2  "Sum3"
  Product2/1 -> Delay5/1
  Delay5/1 -> Add4/2  "K3"
  Add3/1 -> Delay6/1
  Add4/1 -> Delay7/1
  Delay6/1 -> Output_I/1  "Sum4"
  Delay7/1 -> Output_Q/1  "Sum5"
  Input_I/1 -> Add2/1, Add1/1, Delay8/1
  DDS_Q/1 -> Delay11/1, Add/2
  Delay8/1 -> Product/1  "Input_I_w1"
  Delay11/1 -> Product1/2  "DDS_Q_w1"
  Delay9/1 -> Product2/1  "DDS_I_w1"

== system Model/CORE_1_4/DDS_Gen1 ==
  In1 : Inport
  Exp : Math  SaturateOnIntegerOverflow=on
  Gain : Gain  Gain=-1i*2*pi
  Product : Product
  Signal From Workspace1 : dspsrcs4/Signal From Workspace  X=t0  Ts=dt0  nsamps=1  OutputAfterFinalValue=Cyclic repetition  ignoreOrWarnInputAndFrameLengths=off  OutputFrames=off
  Out1 : Outport
  wires:
  Signal From Workspace1/1 -> Gain/1
  Exp/1 -> Out1/1
  Gain/1 -> Product/2
  Product/1 -> Exp/1
  In1/1 -> Product/1

== system Model/CORE_1_4/DDS_Gen2 ==
  In1 : Inport
  Exp : Math  SaturateOnIntegerOverflow=on
  Gain : Gain  Gain=-1i*2*pi
  Product : Product
  Signal From Workspace1 : dspsrcs4/Signal From Workspace  X=t0  Ts=dt0  nsamps=1  OutputAfterFinalValue=Cyclic repetition  ignoreOrWarnInputAndFrameLengths=off  OutputFrames=off
  Out1 : Outport
  wires:
  Signal From Workspace1/1 -> Gain/1
  Exp/1 -> Out1/1
  Gain/1 -> Product/2
  Product/1 -> Exp/1
  In1/1 -> Product/1

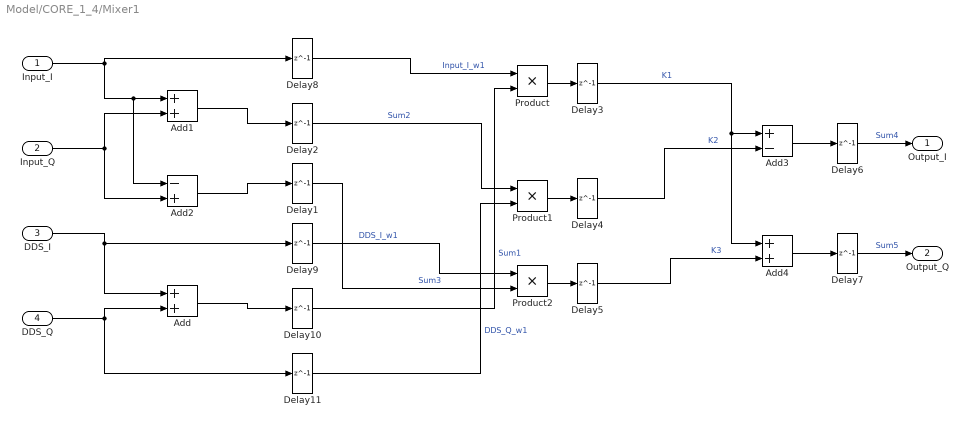
== system Model/CORE_1_4/Mixer1 ==
  Input_I : Inport
  Input_Q : Inport  Port=2
  DDS_I : Inport  Port=3
  DDS_Q : Inport  Port=4
  Add : Sum
  Add1 : Sum
  Add2 : Sum  Inputs=-+
  Add3 : Sum  Inputs=+-
  Add4 : Sum
  Delay{1..11} (11 alike) : Delay  DelayLength=1  InitialCondition=0  SampleTime=dt0
  Product : Product
  Product1 : Product
  Product2 : Product
  Output_I : Outport
  Output_Q : Outport  Port=2
  wires:
  DDS_I/1 -> Delay9/1, Add/1
  Input_Q/1 -> Add2/2, Add1/2
  Add/1 -> Delay10/1
  Delay10/1 -> Product/2  "Sum1"
  Add2/1 -> Delay1/1
  Add1/1 -> Delay2/1
  Product/1 -> Delay3/1
  Delay3/1 -> Add4/1, Add3/1  "K1"
  Delay2/1 -> Product1/1  "Sum2"
  Product1/1 -> Delay4/1
  Delay4/1 -> Add3/2  "K2"
  Delay1/1 -> Product2/2  "Sum3"
  Product2/1 -> Delay5/1
  Delay5/1 -> Add4/2  "K3"
  Add3/1 -> Delay6/1
  Add4/1 -> Delay7/1
  Delay6/1 -> Output_I/1  "Sum4"
  Delay7/1 -> Output_Q/1  "Sum5"
  Input_I/1 -> Add2/1, Add1/1, Delay8/1
  DDS_Q/1 -> Delay11/1, Add/2
  Delay8/1 -> Product/1  "Input_I_w1"
  Delay11/1 -> Product1/2  "DDS_Q_w1"
  Delay9/1 -> Product2/1  "DDS_I_w1"

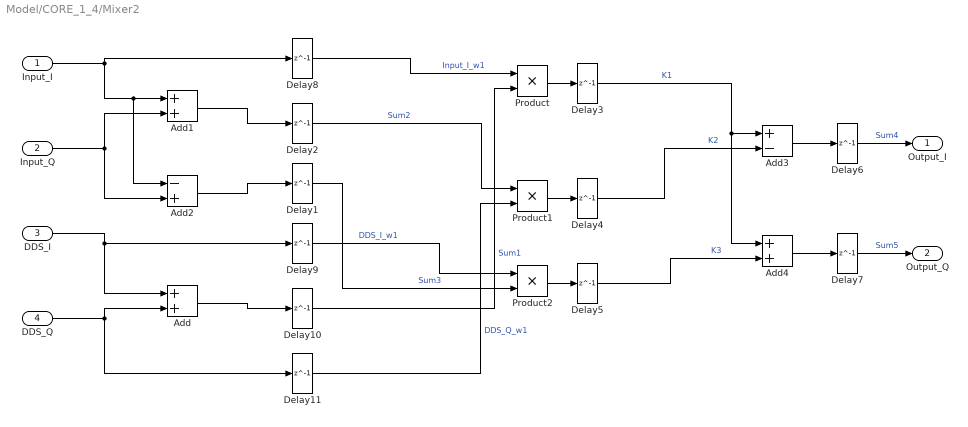
== system Model/CORE_1_4/Mixer2 ==
  Input_I : Inport
  Input_Q : Inport  Port=2
  DDS_I : Inport  Port=3
  DDS_Q : Inport  Port=4
  Add : Sum
  Add1 : Sum
  Add2 : Sum  Inputs=-+
  Add3 : Sum  Inputs=+-
  Add4 : Sum
  Delay{1..11} (11 alike) : Delay  DelayLength=1  InitialCondition=0  SampleTime=dt0
  Product : Product
  Product1 : Product
  Product2 : Product
  Output_I : Outport
  Output_Q : Outport  Port=2
  wires:
  DDS_I/1 -> Delay9/1, Add/1
  Input_Q/1 -> Add2/2, Add1/2
  Add/1 -> Delay10/1
  Delay10/1 -> Product/2  "Sum1"
  Add2/1 -> Delay1/1
  Add1/1 -> Delay2/1
  Product/1 -> Delay3/1
  Delay3/1 -> Add4/1, Add3/1  "K1"
  Delay2/1 -> Product1/1  "Sum2"
  Product1/1 -> Delay4/1
  Delay4/1 -> Add3/2  "K2"
  Delay1/1 -> Product2/2  "Sum3"
  Product2/1 -> Delay5/1
  Delay5/1 -> Add4/2  "K3"
  Add3/1 -> Delay6/1
  Add4/1 -> Delay7/1
  Delay6/1 -> Output_I/1  "Sum4"
  Delay7/1 -> Output_Q/1  "Sum5"
  Input_I/1 -> Add2/1, Add1/1, Delay8/1
  DDS_Q/1 -> Delay11/1, Add/2
  Delay8/1 -> Product/1  "Input_I_w1"
  Delay11/1 -> Product1/2  "DDS_Q_w1"
  Delay9/1 -> Product2/1  "DDS_I_w1"

== system Model/CORE_3_1/Path1 ==
  <IQ> : Inport
  Complex to Real-Imag : ComplexToRealImag
  Complex to Real-Imag1 : ComplexToRealImag
  Constant : Constant  Value=C12  SampleTime=dt0
  DDS_Gen1 : Subsystem
  FIR Dec1 : dspmlti4/FIR Decimation  FilterSource=Input port  h=designMultirateFIR(1,2)  D=2  filtStruct=Direct form  FilterObject=FDECIM  framing=Allow multirate processing  inputOffset=0  outputBufInitCond=0  roundingMode=Floor  overflowMode=off  firstCoeffDataTypeStr=Inherit: Same word length as input  firstCoeffMin=[]  firstCoeffMax=[]  firstCoeffLastDataTypeStr=Inherit: Same word length as input  outputDataTypeStr=Inherit: Same as accumulator  outputMin=[]  outputMax=[]  outputLastDataTypeStr=Inherit: Same as accumulator
  Freq1 : Constant  Value=2.4e6
  Mixer1 : Subsystem
  Real-Imag to Complex : RealImagToComplex
  Out1 : Outport
  wires:
  Constant/1 -> FIR Dec1/2
  Complex to Real-Imag/1 -> Mixer1/1(Input_I)
  Complex to Real-Imag1/1 -> Mixer1/3(DDS_I)
  Mixer1/2(Output_Q) -> Real-Imag to Complex/2
  Freq1/1 -> DDS_Gen1/1(In1)
  Complex to Real-Imag/2 -> Mixer1/2(Input_Q)
  Complex to Real-Imag1/2 -> Mixer1/4(DDS_Q)
  DDS_Gen1/1(Out1) -> Complex to Real-Imag1/1
  Real-Imag to Complex/1 -> FIR Dec1/1
  Mixer1/1(Output_I) -> Real-Imag to Complex/1
  FIR Dec1/1 -> Out1/1
  <IQ>/1 -> Complex to Real-Imag/1

== system Model/CORE_3_1/Path2 ==
  <IQ> : Inport
  Complex to Real-Imag : ComplexToRealImag
  Complex to Real-Imag1 : ComplexToRealImag
  Constant : Constant  Value=C12  SampleTime=dt0
  DDS_Gen1 : Subsystem
  FIR Dec1 : dspmlti4/FIR Decimation  FilterSource=Input port  h=designMultirateFIR(1,2)  D=2  filtStruct=Direct form  FilterObject=FDECIM  framing=Allow multirate processing  inputOffset=0  outputBufInitCond=0  roundingMode=Floor  overflowMode=off  firstCoeffDataTypeStr=Inherit: Same word length as input  firstCoeffMin=[]  firstCoeffMax=[]  firstCoeffLastDataTypeStr=Inherit: Same word length as input  outputDataTypeStr=Inherit: Same as accumulator  outputMin=[]  outputMax=[]  outputLastDataTypeStr=Inherit: Same as accumulator
  Freq1 : Constant  Value=2.4e6
  Mixer1 : Subsystem
  Real-Imag to Complex : RealImagToComplex
  Out1 : Outport
  wires:
  Constant/1 -> FIR Dec1/2
  Complex to Real-Imag/1 -> Mixer1/1(Input_I)
  Complex to Real-Imag1/1 -> Mixer1/3(DDS_I)
  Mixer1/2(Output_Q) -> Real-Imag to Complex/2
  Freq1/1 -> DDS_Gen1/1(In1)
  Complex to Real-Imag/2 -> Mixer1/2(Input_Q)
  Complex to Real-Imag1/2 -> Mixer1/4(DDS_Q)
  DDS_Gen1/1(Out1) -> Complex to Real-Imag1/1
  Real-Imag to Complex/1 -> FIR Dec1/1
  Mixer1/1(Output_I) -> Real-Imag to Complex/1
  FIR Dec1/1 -> Out1/1
  <IQ>/1 -> Complex to Real-Imag/1

== system Model/CORE_3_1/Path3 ==
  <IQ> : Inport
  Complex to Real-Imag : ComplexToRealImag
  Complex to Real-Imag1 : ComplexToRealImag
  Constant : Constant  Value=C12  SampleTime=dt0
  DDS_Gen1 : Subsystem
  FIR Dec1 : dspmlti4/FIR Decimation  FilterSource=Input port  h=designMultirateFIR(1,2)  D=2  filtStruct=Direct form  FilterObject=FDECIM  framing=Allow multirate processing  inputOffset=0  outputBufInitCond=0  roundingMode=Floor  overflowMode=off  firstCoeffDataTypeStr=Inherit: Same word length as input  firstCoeffMin=[]  firstCoeffMax=[]  firstCoeffLastDataTypeStr=Inherit: Same word length as input  outputDataTypeStr=Inherit: Same as accumulator  outputMin=[]  outputMax=[]  outputLastDataTypeStr=Inherit: Same as accumulator
  Freq1 : Constant  Value=2.4e6
  Mixer1 : Subsystem
  Real-Imag to Complex : RealImagToComplex
  Out1 : Outport
  wires:
  Constant/1 -> FIR Dec1/2
  Complex to Real-Imag/1 -> Mixer1/1(Input_I)
  Complex to Real-Imag1/1 -> Mixer1/3(DDS_I)
  Mixer1/2(Output_Q) -> Real-Imag to Complex/2
  Freq1/1 -> DDS_Gen1/1(In1)
  Complex to Real-Imag/2 -> Mixer1/2(Input_Q)
  Complex to Real-Imag1/2 -> Mixer1/4(DDS_Q)
  DDS_Gen1/1(Out1) -> Complex to Real-Imag1/1
  Real-Imag to Complex/1 -> FIR Dec1/1
  Mixer1/1(Output_I) -> Real-Imag to Complex/1
  FIR Dec1/1 -> Out1/1
  <IQ>/1 -> Complex to Real-Imag/1

== system Model/CORE_3_1/Path4 ==
  <IQ> : Inport
  Complex to Real-Imag : ComplexToRealImag
  Complex to Real-Imag1 : ComplexToRealImag
  Constant : Constant  Value=C12  SampleTime=dt0
  DDS_Gen1 : Subsystem
  FIR Dec1 : dspmlti4/FIR Decimation  FilterSource=Input port  h=designMultirateFIR(1,2)  D=2  filtStruct=Direct form  FilterObject=FDECIM  framing=Allow multirate processing  inputOffset=0  outputBufInitCond=0  roundingMode=Floor  overflowMode=off  firstCoeffDataTypeStr=Inherit: Same word length as input  firstCoeffMin=[]  firstCoeffMax=[]  firstCoeffLastDataTypeStr=Inherit: Same word length as input  outputDataTypeStr=Inherit: Same as accumulator  outputMin=[]  outputMax=[]  outputLastDataTypeStr=Inherit: Same as accumulator
  Freq1 : Constant  Value=2.4e6
  Mixer1 : Subsystem
  Real-Imag to Complex : RealImagToComplex
  Out1 : Outport
  wires:
  Constant/1 -> FIR Dec1/2
  Complex to Real-Imag/1 -> Mixer1/1(Input_I)
  Complex to Real-Imag1/1 -> Mixer1/3(DDS_I)
  Mixer1/2(Output_Q) -> Real-Imag to Complex/2
  Freq1/1 -> DDS_Gen1/1(In1)
  Complex to Real-Imag/2 -> Mixer1/2(Input_Q)
  Complex to Real-Imag1/2 -> Mixer1/4(DDS_Q)
  DDS_Gen1/1(Out1) -> Complex to Real-Imag1/1
  Real-Imag to Complex/1 -> FIR Dec1/1
  Mixer1/1(Output_I) -> Real-Imag to Complex/1
  FIR Dec1/1 -> Out1/1
  <IQ>/1 -> Complex to Real-Imag/1

== system Model/CORE_3_1/Path5 ==
  <IQ> : Inport
  Complex to Real-Imag : ComplexToRealImag
  Complex to Real-Imag1 : ComplexToRealImag
  Constant : Constant  Value=C12  SampleTime=dt0
  DDS_Gen1 : Subsystem
  FIR Dec1 : dspmlti4/FIR Decimation  FilterSource=Input port  h=designMultirateFIR(1,2)  D=2  filtStruct=Direct form  FilterObject=FDECIM  framing=Allow multirate processing  inputOffset=0  outputBufInitCond=0  roundingMode=Floor  overflowMode=off  firstCoeffDataTypeStr=Inherit: Same word length as input  firstCoeffMin=[]  firstCoeffMax=[]  firstCoeffLastDataTypeStr=Inherit: Same word length as input  outputDataTypeStr=Inherit: Same as accumulator  outputMin=[]  outputMax=[]  outputLastDataTypeStr=Inherit: Same as accumulator
  Freq1 : Constant  Value=2.4e6
  Mixer1 : Subsystem
  Real-Imag to Complex : RealImagToComplex
  Out1 : Outport
  wires:
  Constant/1 -> FIR Dec1/2
  Complex to Real-Imag/1 -> Mixer1/1(Input_I)
  Complex to Real-Imag1/1 -> Mixer1/3(DDS_I)
  Mixer1/2(Output_Q) -> Real-Imag to Complex/2
  Freq1/1 -> DDS_Gen1/1(In1)
  Complex to Real-Imag/2 -> Mixer1/2(Input_Q)
  Complex to Real-Imag1/2 -> Mixer1/4(DDS_Q)
  DDS_Gen1/1(Out1) -> Complex to Real-Imag1/1
  Real-Imag to Complex/1 -> FIR Dec1/1
  Mixer1/1(Output_I) -> Real-Imag to Complex/1
  FIR Dec1/1 -> Out1/1
  <IQ>/1 -> Complex to Real-Imag/1

== system Model/CORE_3_1/Path6 ==
  <IQ> : Inport
  Complex to Real-Imag : ComplexToRealImag
  Complex to Real-Imag1 : ComplexToRealImag
  Constant : Constant  Value=C12  SampleTime=dt0
  DDS_Gen1 : Subsystem
  FIR Dec1 : dspmlti4/FIR Decimation  FilterSource=Input port  h=designMultirateFIR(1,2)  D=2  filtStruct=Direct form  FilterObject=FDECIM  framing=Allow multirate processing  inputOffset=0  outputBufInitCond=0  roundingMode=Floor  overflowMode=off  firstCoeffDataTypeStr=Inherit: Same word length as input  firstCoeffMin=[]  firstCoeffMax=[]  firstCoeffLastDataTypeStr=Inherit: Same word length as input  outputDataTypeStr=Inherit: Same as accumulator  outputMin=[]  outputMax=[]  outputLastDataTypeStr=Inherit: Same as accumulator
  Freq1 : Constant  Value=2.4e6
  Mixer1 : Subsystem
  Real-Imag to Complex : RealImagToComplex
  Out1 : Outport
  wires:
  Constant/1 -> FIR Dec1/2
  Complex to Real-Imag/1 -> Mixer1/1(Input_I)
  Complex to Real-Imag1/1 -> Mixer1/3(DDS_I)
  Mixer1/2(Output_Q) -> Real-Imag to Complex/2
  Freq1/1 -> DDS_Gen1/1(In1)
  Complex to Real-Imag/2 -> Mixer1/2(Input_Q)
  Complex to Real-Imag1/2 -> Mixer1/4(DDS_Q)
  DDS_Gen1/1(Out1) -> Complex to Real-Imag1/1
  Real-Imag to Complex/1 -> FIR Dec1/1
  Mixer1/1(Output_I) -> Real-Imag to Complex/1
  FIR Dec1/1 -> Out1/1
  <IQ>/1 -> Complex to Real-Imag/1

== system Model/CORE_3_1/Path7 ==
  <IQ> : Inport
  Complex to Real-Imag : ComplexToRealImag
  Complex to Real-Imag1 : ComplexToRealImag
  Constant : Constant  Value=C12  SampleTime=dt0
  DDS_Gen1 : Subsystem
  FIR Dec1 : dspmlti4/FIR Decimation  FilterSource=Input port  h=designMultirateFIR(1,2)  D=2  filtStruct=Direct form  FilterObject=FDECIM  framing=Allow multirate processing  inputOffset=0  outputBufInitCond=0  roundingMode=Floor  overflowMode=off  firstCoeffDataTypeStr=Inherit: Same word length as input  firstCoeffMin=[]  firstCoeffMax=[]  firstCoeffLastDataTypeStr=Inherit: Same word length as input  outputDataTypeStr=Inherit: Same as accumulator  outputMin=[]  outputMax=[]  outputLastDataTypeStr=Inherit: Same as accumulator
  Freq1 : Constant  Value=2.4e6
  Mixer1 : Subsystem
  Real-Imag to Complex : RealImagToComplex
  Out1 : Outport
  wires:
  Constant/1 -> FIR Dec1/2
  Complex to Real-Imag/1 -> Mixer1/1(Input_I)
  Complex to Real-Imag1/1 -> Mixer1/3(DDS_I)
  Mixer1/2(Output_Q) -> Real-Imag to Complex/2
  Freq1/1 -> DDS_Gen1/1(In1)
  Complex to Real-Imag/2 -> Mixer1/2(Input_Q)
  Complex to Real-Imag1/2 -> Mixer1/4(DDS_Q)
  DDS_Gen1/1(Out1) -> Complex to Real-Imag1/1
  Real-Imag to Complex/1 -> FIR Dec1/1
  Mixer1/1(Output_I) -> Real-Imag to Complex/1
  FIR Dec1/1 -> Out1/1
  <IQ>/1 -> Complex to Real-Imag/1
